simulink model "AccelerationControlSysIdentification"  (R2018a)
settings: Solver=FixedStepAuto  StartTime=0.0  StopTime=inf  RelTol=1e-3  EnableMultiTasking=on
libraries: simulink x15, simulink_extras x1, raspberrypilib x1
settings Model: SimulationMode=external  Creator=Paul  LastModifiedBy=domin
settings SolverCC: PositivePriorityOrder=on
settings OptimizationCC: PassReuseOutputArgsThreshold=0  MaxStackSize=64
settings DebuggingCC: ParameterOverflowMsg=warning  ParameterTunabilityLossMsg=error
settings HardwareCC: ProdBitPerPointer=32  ProdBitPerSizeT=32  ProdBitPerPtrDiffT=32  ProdLargestAtomicInteger=Long  ProdLargestAtomicFloat=Double  ProdWordSize=32  ProdHWDeviceType=ARM Compatible->ARM Cortex  UseEmbeddedCoderFeatures=off
settings SFSimCC: MATLABDynamicMemAlloc=off
settings RTWCC: SystemTargetFile=ert.tlc  HardwareBoard=Raspberry Pi  TLCOptions="-aInlineSetEventsForThisBaseRateFcn=TLC_FALSE -aSuppressMultiTaskScheduler=TLC_FALSE  -aRateBasedStepFcn=0"  TemplateMakefile=ert_default_tmf  GenerateReport=on  Toolchain=GNU GCC Raspberry Pi  LaunchReport=on
settings CodeAppCC: ForceParamTrailComments=on  OperatorAnnotations=on  StateflowObjectComments=on  MATLABSourceComments=on
settings ERTTargetCC: ERTCustomFileBanners=off  SupportContinuousTime=on  SupportNonInlinedSFcns=on  RemoveResetFunc=off  SupportVariableSizeSignals=on  ModelStepFunctionPrototypeControlCompliant=off

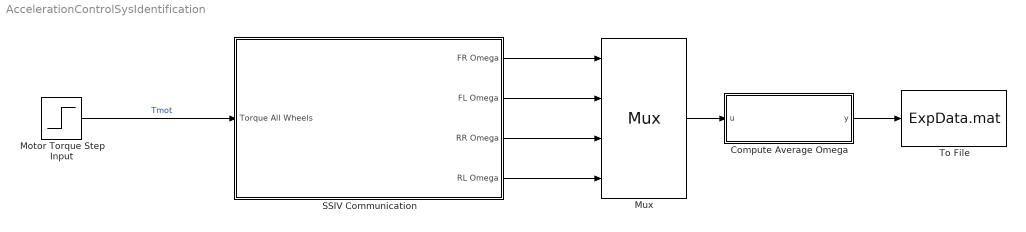
== system AccelerationControlSysIdentification ==
  Compute Average Omega : MATLAB Function  TreatAsAtomicUnit=on
  "Motor Torque Step Input " : Step  SampleTime=0
  Mux : Mux
      settings: DisplayOption=signals
  SSIV Communication : Subsystem
  To File : ToFile  Filename=ExpData.mat  SaveFormat=Timeseries
  wires:
  "Motor Torque Step Input "/1 -> SSIV Communication/1(Torque All Wheels)  "Tmot"
  Compute Average Omega/1(y) -> To File/1
  SSIV Communication/1(FR Omega) -> Mux/1
  SSIV Communication/2(FL Omega) -> Mux/2
  SSIV Communication/3(RR Omega) -> Mux/3
  SSIV Communication/4(RL Omega) -> Mux/4
  Mux/1 -> Compute Average Omega/1(u)

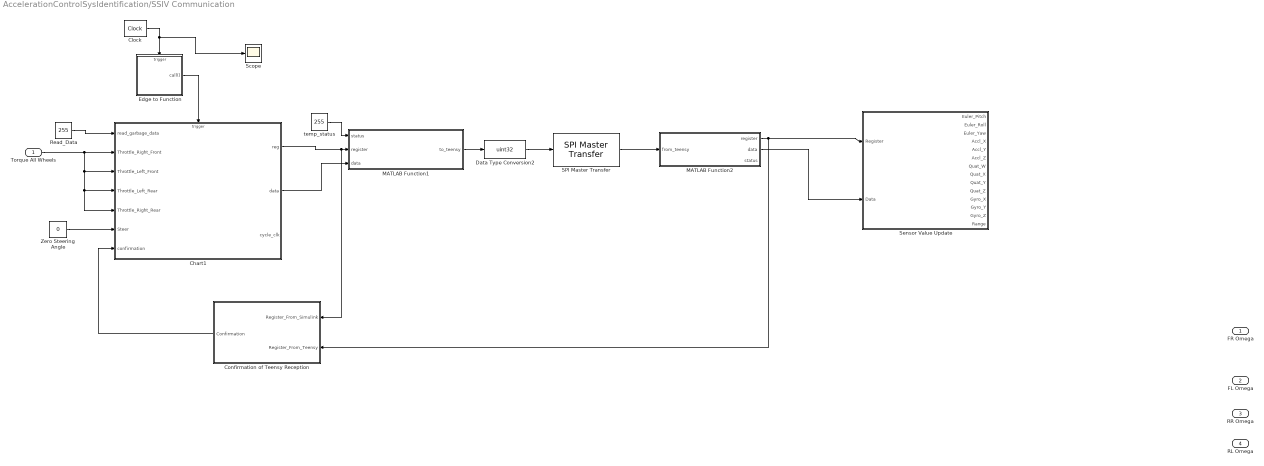
== system AccelerationControlSysIdentification/SSIV Communication ==
  Torque All Wheels : Inport
  Chart1 : Stateflow chart  TreatAsAtomicUnit=on
  Clock : simulink_extras/Flip Flops/Clock  period=.005
  Confirmation of Teensy Reception : Subsystem
  Data Type Conversion2 : DataTypeConversion  OutDataTypeStr=uint32
  "Edge to Function " : Stateflow chart  TreatAsAtomicUnit=on
  MATLAB Function1 : MATLAB Function  TreatAsAtomicUnit=on
  MATLAB Function2 : MATLAB Function  TreatAsAtomicUnit=on
  Read_Data : Constant  Value=255
  SPI Master Transfer : raspberrypilib/SPI Master Transfer  BoardProperty=Pi 3 Model B  SPIModule=uint32(0)  Mode=Master  BusSpeed=1000000  Pin=SPI0_CE1  FirstBitToTransfer=Most significant bit (MSB)  ClockMode=0  BlockFunction=Transfer  RegisterAddress=0  OutputDataType=int8  OutputDataLength=1
      settings: SourceProductName=Simulink Support Package for Raspberry Pi Hardware  SourceProductBaseCode=RASPPI
  Scope : Scope
  Sensor Value Update : Subsystem
  Zero Steering Angle : Constant  Value=0
  temp_status : Constant  Value=255
  FR Omega : Outport
  FL Omega : Outport  Port=2
  RR Omega : Outport  Port=3
  RL Omega : Outport  Port=4
  wires:
  Clock/1 -> Scope/1, "Edge to Function "/Trigger
  Chart1/1(reg) -> Confirmation of Teensy Reception/1(Register_From_Simulink), MATLAB Function1/2(register)
  Data Type Conversion2/1 -> SPI Master Transfer/1
  temp_status/1 -> MATLAB Function1/1(status)
  SPI Master Transfer/1 -> MATLAB Function2/1(from_teensy)
  MATLAB Function1/1(to_teensy) -> Data Type Conversion2/1
  Chart1/2(data) -> MATLAB Function1/3(data)
  "Edge to Function "/1(call()) -> Chart1/Trigger
  MATLAB Function2/2(data) -> Sensor Value Update/2(Data)
  Read_Data/1 -> Chart1/1(read_garbage_data)
  MATLAB Function2/1(register) -> Confirmation of Teensy Reception/2(Register_From_Teensy), Sensor Value Update/1(Register)
  Confirmation of Teensy Reception/1(Confirmation) -> Chart1/7(confirmation)
  Torque All Wheels/1 -> Chart1/2(Throttle_Right_Front), Chart1/5(Throttle_Right_Rear), Chart1/4(Throttle_Left_Rear), Chart1/3(Throttle_Left_Front)
  ? -> FR Omega/1
  Zero Steering Angle/1 -> Chart1/6(Steer)

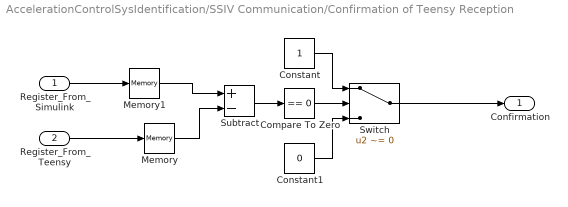
== system AccelerationControlSysIdentification/SSIV Communication/Confirmation of Teensy Reception ==
  Register_From_Simulink : Inport
  Register_From_Teensy : Inport  Port=2
  Compare To Zero : simulink/Logic and Bit Operations/Compare To Zero  relop===  OutDataTypeStr=boolean
  Constant : Constant
  Constant1 : Constant  Value=0
  Memory : Memory
  Memory1 : Memory
  Subtract : Sum  Inputs=+-
  Switch : Switch  Criteria=u2 ~= 0
  Confirmation : Outport
  wires:
  Subtract/1 -> Compare To Zero/1
  Constant1/1 -> Switch/3
  Compare To Zero/1 -> Switch/2
  Constant/1 -> Switch/1
  Switch/1 -> Confirmation/1
  Register_From_Simulink/1 -> Memory1/1
  Register_From_Teensy/1 -> Memory/1
  Memory/1 -> Subtract/2
  Memory1/1 -> Subtract/1

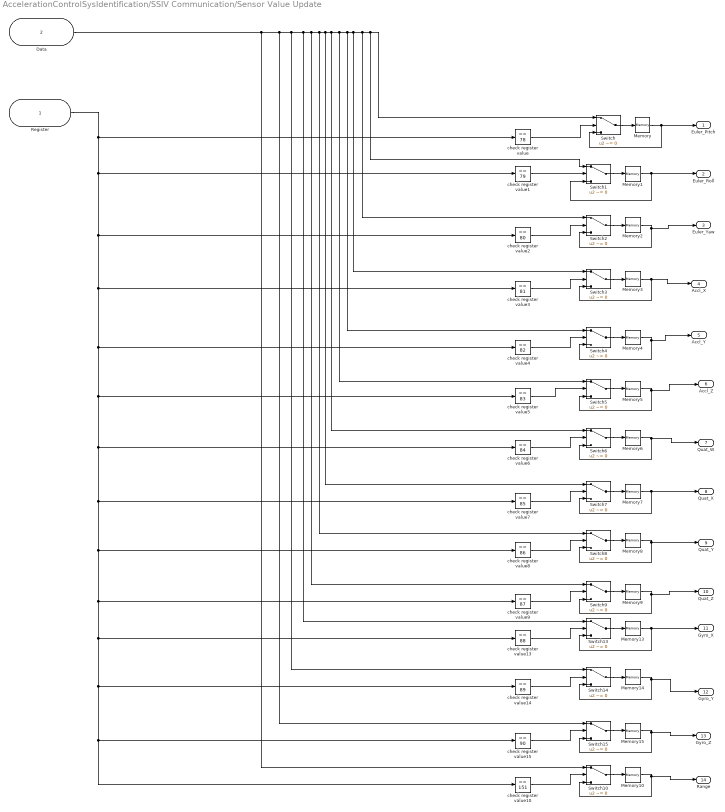
== system AccelerationControlSysIdentification/SSIV Communication/Sensor Value Update ==
  Register : Inport
  Data : Inport  Port=2
  Memory{,1..10,13..15} (14 alike) : Memory
  Switch{,1..10,13..15} (14 alike) : Switch  Criteria=u2 ~= 0
  check register value : simulink/Logic and Bit Operations/Compare To Constant  relop===  const=78  OutDataTypeStr=boolean
  check register value1 : simulink/Logic and Bit Operations/Compare To Constant  relop===  const=79  OutDataTypeStr=boolean
  check register value10 : simulink/Logic and Bit Operations/Compare To Constant  relop===  const=151  OutDataTypeStr=boolean
  check register value13 : simulink/Logic and Bit Operations/Compare To Constant  relop===  const=88  OutDataTypeStr=boolean
  check register value14 : simulink/Logic and Bit Operations/Compare To Constant  relop===  const=89  OutDataTypeStr=boolean
  check register value15 : simulink/Logic and Bit Operations/Compare To Constant  relop===  const=90  OutDataTypeStr=boolean
  check register value2 : simulink/Logic and Bit Operations/Compare To Constant  relop===  const=80  OutDataTypeStr=boolean
  check register value3 : simulink/Logic and Bit Operations/Compare To Constant  relop===  const=81  OutDataTypeStr=boolean
  check register value4 : simulink/Logic and Bit Operations/Compare To Constant  relop===  const=82  OutDataTypeStr=boolean
  check register value5 : simulink/Logic and Bit Operations/Compare To Constant  relop===  const=83  OutDataTypeStr=boolean
  check register value6 : simulink/Logic and Bit Operations/Compare To Constant  relop===  const=84  OutDataTypeStr=boolean
  check register value7 : simulink/Logic and Bit Operations/Compare To Constant  relop===  const=85  OutDataTypeStr=boolean
  check register value8 : simulink/Logic and Bit Operations/Compare To Constant  relop===  const=86  OutDataTypeStr=boolean
  check register value9 : simulink/Logic and Bit Operations/Compare To Constant  relop===  const=87  OutDataTypeStr=boolean
  Euler_Pitch : Outport
  Euler_Roll : Outport  Port=2
  Euler_Yaw : Outport  Port=3
  Accl_X : Outport  Port=4
  Accl_Y : Outport  Port=5
  Accl_Z : Outport  Port=6
  Quat_W : Outport  Port=7
  Quat_X : Outport  Port=8
  Quat_Y : Outport  Port=9
  Quat_Z : Outport  Port=10
  Gyro_X : Outport  Port=11
  Gyro_Y : Outport  Port=12
  Gyro_Z : Outport  Port=13
  Range : Outport  Port=14
  wires:
  Memory6/1 -> Quat_W/1, Switch6/3
  Memory5/1 -> Accl_Z/1, Switch5/3
  check register value14/1 -> Switch14/2
  Switch14/1 -> Memory14/1
  check register value3/1 -> Switch3/2
  Switch1/1 -> Memory1/1
  Memory4/1 -> Accl_Y/1, Switch4/3
  check register value4/1 -> Switch4/2
  check register value2/1 -> Switch2/2
  Switch3/1 -> Memory3/1
  Switch6/1 -> Memory6/1
  Switch2/1 -> Memory2/1
  Switch9/1 -> Memory9/1
  Memory14/1 -> Gyro_Y/1, Switch14/3
  Memory/1 -> Euler_Pitch/1, Switch/3
  Switch13/1 -> Memory13/1
  Memory1/1 -> Euler_Roll/1, Switch1/3
  check register value6/1 -> Switch6/2
  Switch4/1 -> Memory4/1
  check register value1/1 -> Switch1/2
  Memory3/1 -> Accl_X/1, Switch3/3
  check register value/1 -> Switch/2
  Switch8/1 -> Memory8/1
  Memory9/1 -> Quat_Z/1, Switch9/3
  Switch/1 -> Memory/1
  Memory2/1 -> Euler_Yaw/1, Switch2/3
  Memory8/1 -> Quat_Y/1, Switch8/3
  Memory7/1 -> Quat_X/1, Switch7/3
  check register value13/1 -> Switch13/2
  Switch15/1 -> Memory15/1
  check register value7/1 -> Switch7/2
  check register value15/1 -> Switch15/2
  Memory13/1 -> Gyro_X/1, Switch13/3
  Memory15/1 -> Gyro_Z/1, Switch15/3
  check register value8/1 -> Switch8/2
  Switch7/1 -> Memory7/1
  check register value5/1 -> Switch5/2
  check register value9/1 -> Switch9/2
  Switch5/1 -> Memory5/1
  Register/1 -> check register value/1, check register value1/1, check register value3/1, check register value4/1, check register value6/1, check register value7/1, check register value8/1, check register value9/1, check register value13/1, check register value10/1, check register value15/1, check register value14/1, check register value5/1, check register value2/1
  Memory10/1 -> Range/1, Switch10/3
  Data/1 -> Switch10/1, Switch15/1, Switch14/1, Switch13/1, Switch9/1, Switch8/1, Switch7/1, Switch6/1, Switch5/1, Switch4/1, Switch3/1, Switch2/1, Switch1/1, Switch/1
  check register value10/1 -> Switch10/2
  Switch10/1 -> Memory10/1

== matlab function AccelerationControlSysIdentification/SSIV Communication/MATLAB Function1 ==
  data: status input; register input; to_teensy output; data input
function to_teensy = input_of_spi_master_transfer(status,register,data)
% to_teensy is a uint32 data type
% The following mathematical operation makes the status input be the
%   1st byte of to_teensy, register input the 2nd byte and
%   data input the last two bytes of to_teensy.
% data input is added by 500 to keep the value unsigned data is a
% value between -500 and 500.  The 500 is subtracted back out on the Teensy
% end.
%% output variables
status_output=0;
register_output=0;
data_output=0;
%% adjust status input value so that the value can be represented as uint8
if (status>255)
    status_output=255;
elseif (status<0)
    status_output=0;
else
    status_output=status;
end
%% adjust register input value so that the value can be represented as uint8
if (register>255)
    register_output=255;
elseif (register<0)
    register_output=0;
else
    register_output=register;
end
%% adjust data input value so that the value can be represented as uint16
if (data>65035) %uint16 max value - 500
    data_output=65035;
elseif (data<-500)
    data_output=-500;
else
    data_output=data;
end
%% output
to_teensy = 16777216*(status_output)+65536*(register_output)+1*(data_output+500);

== stateflow chart AccelerationControlSysIdentification/SSIV Communication/Edge to Function  ==
  (default) -> (junction 2) : {call;}
  events: edge input RISING_EDGE_EVENT; call output FUNCTION_CALL_EVENT

== matlab function AccelerationControlSysIdentification/SSIV Communication/MATLAB Function2 ==
  data: register output; from_teensy input; data output; status output
function [register,data,status] = output_of_spi_master_transfer(from_teensy)
%% from_teensy data format (uint32)
%status is first byte of 1st byte
%register is second byte of 2nd byte
%high byte of teensy data is 3rd byte
%low byte of teensy data is 4th byte

%% create blank variables to be filled with 1 or 2 bytes of data
data_hex = blanks(4);     
register_hex = blanks(2);
status_hex = blanks(2);

%% convert from_teensy to hex
hex_input = dec2hex(from_teensy,8);

%% fill up status with 2st byte of hex_input
status_hex(1) = hex_input(1);
status_hex(2) = hex_input(2);

%% fill up register with 2nd byte of hex_input
register_hex(1) = hex_input(3);
register_hex(2) = hex_input(4);

%% fill up data with last 2 bytes of hex_input
data_hex(1) = hex_input(5);
data_hex(2) = hex_input(6);
data_hex(3) = hex_input(7);
data_hex(4) = hex_input(8);

%% convert the hex values back to decimal and output
register = hex2dec(register_hex);
if (register == 151)
    data = (hex2dec(data_hex))-500;
else    
    data = (hex2dec(data_hex)/100)-500;
end 
status  = hex2dec(status_hex);

end

== matlab function AccelerationControlSysIdentification/Compute Average Omega ==
  data: u input; y output
function y = WheelAverageSpeed(u)

OmegaAVG = mean(u(1),u(2),u(3),u(4));

y = OmegaAVG;

== stateflow chart AccelerationControlSysIdentification/SSIV Communication/Chart1 ==
  settings: executeAtInitialization=1
  state Range_finder
    entry: reg=151;
    entry: data = read_garbage_data;
    entry: cycle_clk = 0; %
    i= 0;
  state Steering_Write
    entry: reg = 121;
    entry: data = Steer;
    entry: cycle_clk = 0; %
    i = 1;
  state Throttle_Left_Rear_Write [commented out]
    entry: reg=104;
    entry: data = Throttle_Left_Rear;
    entry: cycle_clk = 0; %
    i= 2;
  state Throttle_Right_Rear_Write [commented out]
    entry: reg=103;
    entry: data = Throttle_Right_Rear;
    entry: cycle_clk = 0; %
    i= 3;
  state Gyro_Z_Read [commented out]
    entry: reg=90;
    entry: data = read_garbage_data;
    entry: cycle_clk = 0; %
    i= 18;
  state Throttle_Left_Front_Write [commented out]
    entry: reg=102;
    entry: data = Throttle_Left_Front;
    entry: cycle_clk = 0; %
    i= 4;
  state Gyro_Y_Read [commented out]
    entry: reg=89;
    entry: data = read_garbage_data;
    entry: cycle_clk = 0; %
    i= 17;
  state Throttle_Right_Front_Write [commented out]
    entry: reg = 101;
    entry: data = Throttle_Right_Front;
    entry: cycle_clk = 0; %
    i = 5;
  state Throttle_All_Write
    entry: reg = 100;
    entry: data = Throttle_Right_Front;
    entry: cycle_clk = 0; %
    i = 6;
  state Gyro_X_Read [commented out]
    entry: reg=88;
    entry: data = read_garbage_data;
    entry: cycle_clk = 0; %
    i= 16;
  state Accl_X_Read [commented out]
    entry: reg=81;
    entry: data = read_garbage_data;
    entry: cycle_clk = 1; %
    i= 6;
  state Quaternion_Z_Read [commented out]
    entry: reg=87;
    entry: data = read_garbage_data;
    entry: cycle_clk = 0; %
    i= 15;
  state Accl_Y_Read [commented out]
    entry: reg=82;
    i= i + 1;
    entry: data = read_garbage_data;
    entry: cycle_clk = 0; %
    i= 7;
  state Quaternion_Y_Read [commented out]
    entry: reg=86;
    entry: data = read_garbage_data;
    entry: cycle_clk = 0; %
    i= 14;
  state Accl_Z_Read [commented out]
    entry: reg=83;
    entry: data = read_garbage_data;
    entry: cycle_clk = 0; %
    i= 8;
  state Quaternion_X_Read [commented out]
    entry: reg=85;
    entry: data = read_garbage_data;
    entry: cycle_clk = 0; %
    i= 13;
  state Quaternion_W_Read [commented out]
    entry: reg=84;
    entry: data = read_garbage_data;
    entry: cycle_clk = 0; %
    i= 12;
  state Euler_Yaw_Read [commented out]
    entry: reg=80;
    entry: data = read_garbage_data;
    entry: cycle_clk = 0; %
    i = 9;
  state Euler_Roll_Read [commented out]
    entry: reg=79;
    entry: data = read_garbage_data;
    entry: cycle_clk = 0; %
    i= 10;
  state Euler_Pitch_Read [commented out]
    entry: reg=78;
    entry: data = read_garbage_data;
    entry: cycle_clk = 0; %
    i= 11;
  (default) -> Steering_Write : {i=0;}
  Range_finder -> Steering_Write : [confirmation==1 & i==0]
  Gyro_Z_Read -> ? [commented out] : [confirmation==1 & i==18]
  (default) -> Throttle_Left_Rear_Write [commented out] : [confirmation==1 & i==1]
  Steering_Write -> Throttle_All_Write : [confirmation==1 & i==1]
  Throttle_Left_Rear_Write -> Throttle_Right_Rear_Write [commented out] : [confirmation==1 & i==2]
  Throttle_All_Write -> Range_finder : [confirmation==1 & i==6]
  Gyro_Y_Read -> Gyro_Z_Read [commented out] : [confirmation==1 & i==17]
  Throttle_Right_Rear_Write -> Throttle_Left_Front_Write [commented out] : [confirmation==1 & i==3]
  Throttle_Left_Front_Write -> Throttle_Right_Front_Write [commented out] : [confirmation==1 & i==4]
  Gyro_X_Read -> Gyro_Y_Read [commented out] : [confirmation==1 & i==16]
  Quaternion_Z_Read -> Gyro_X_Read [commented out] : [confirmation==1 & i==15]
  Quaternion_Y_Read -> Quaternion_Z_Read [commented out] : [confirmation==1 & i==14]
  Accl_X_Read -> Accl_Y_Read [commented out] : [confirmation==1 & i==6]
  Quaternion_X_Read -> Quaternion_Y_Read [commented out] : [confirmation==1 & i==13]
  Accl_Y_Read -> Accl_Z_Read [commented out] : [confirmation==1 & i==7]
  Quaternion_W_Read -> Quaternion_X_Read [commented out] : [confirmation==1 & i==12]
  Accl_Z_Read -> Euler_Yaw_Read [commented out] : [confirmation==1 & i==8]
  Euler_Yaw_Read -> Euler_Roll_Read [commented out] : [confirmation==1 & i==9]
  Euler_Pitch_Read -> Quaternion_W_Read [commented out] : [confirmation==1 & i==11]
  Euler_Roll_Read -> Euler_Pitch_Read [commented out] : [confirmation==1 & i==10]
  data: i local; reg output; data output; read_garbage_data input; Throttle_Right_Front input; Throttle_Left_Front input; Throttle_Left_Rear input; Throttle_Right_Rear input; Steer input; confirmation input; cycle_clk output
  events: Call input FUNCTION_CALL_EVENT
